simulink subsystem "Doublet"  (R2025a)
settings: Solver=VariableStepAuto  StartTime=0.0  StopTime=10.0  RelTol=1e-3
settings Model: Creator=17036  LastModifiedBy=gurt1

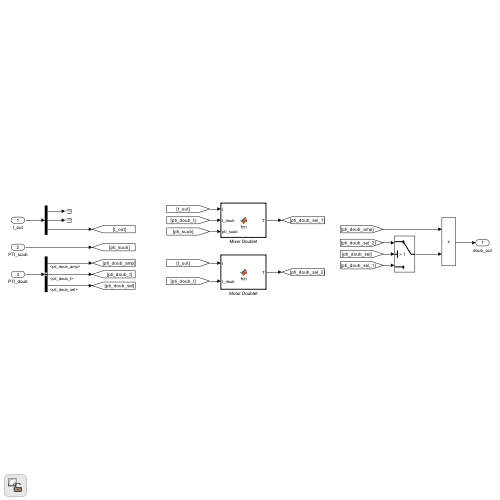
[thumbnail: Simulink's stored preview of the top-level diagram]
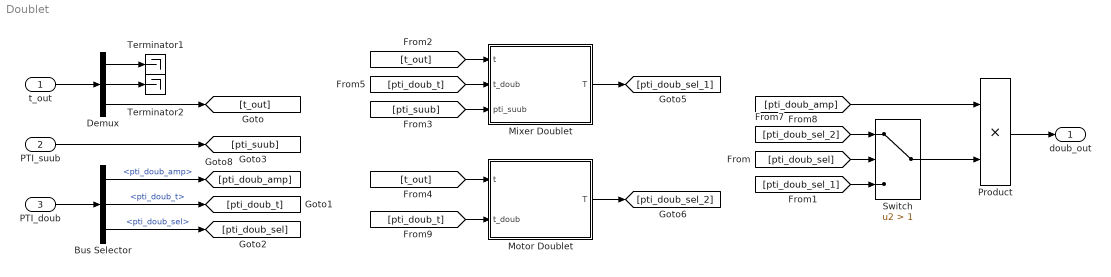
== system Doublet ==
  t_out : Inport
  PTI_suub : Inport  Port=2
  PTI_doub : Inport  Port=3
  Bus Selector : BusSelector  OutputSignals=pti_doub_amp,pti_doub_t,pti_doub_sel
  Demux : Demux  Outputs=3
  Mixer Doublet : MATLAB Function  TreatAsAtomicUnit=on
  Motor Doublet : MATLAB Function  TreatAsAtomicUnit=on
  Product : Product
  Switch : Switch  Criteria=u2 > Threshold  Threshold=1  SaturateOnIntegerOverflow=off  InputSameDT=off
  Terminator1 : Terminator
  Terminator2 : Terminator
  doub_out : Outport
  wires:
  PTI_doub/1 -> Bus Selector/1
  Bus Selector/1 -> [pti_doub_amp]  "<pti_doub_amp>"
  Bus Selector/2 -> [pti_doub_t]  "<pti_doub_t>"
  Bus Selector/3 -> [pti_doub_sel]  "<pti_doub_sel>"
  [pti_doub_sel] -> Switch/2
  Mixer Doublet/1(T) -> [pti_doub_sel_1]
  [t_out] -> Mixer Doublet/1(t)
  Switch/1 -> Product/2
  [pti_doub_amp] -> Product/1
  Product/1 -> doub_out/1
  t_out/1 -> Demux/1
  Motor Doublet/1(T) -> [pti_doub_sel_2]
  PTI_suub/1 -> [pti_suub]
  [pti_doub_t] -> Mixer Doublet/2(t_doub)
  [pti_suub] -> Mixer Doublet/3(pti_suub)
  [pti_doub_t] -> Motor Doublet/2(t_doub)
  [t_out] -> Motor Doublet/1(t)
  Demux/2 -> Terminator2/1
  [pti_doub_sel_2] -> Switch/1
  [pti_doub_sel_1] -> Switch/3
  Demux/3 -> [t_out]
  Demux/1 -> Terminator1/1

== matlab function Doublet/Mixer Doublet ==
  data: t input; T output; t_doub input; pti_suub input
function T = fcn(t, t_doub, pti_suub)

% Roll, Pitch, Yaw, Thrust

% Mixing matrix for quadcopter control (roll, pitch, yaw, throttle)
M = [-1  1 -1 1;
      1 -1 -1 1;
      1  1  1 1;
     -1 -1  1 1];

% Select the column corresponding to the axis mode
axis_mode = M(:,pti_suub+1);

% Calculate the total duration of one full 1-2-1 doublet cycle
cycle_t = 4 * t_doub;

% Find the current time within the current cycle
% current_cycle_t = mod(t, cycle_t);

% Determine the control input based on the time within the cycle
if t>0

if t < t_doub
    % First 1x input
    T = axis_mode;
elseif t < 3 * t_doub
    % 2x input
    T = -1 .* axis_mode;
elseif t < 4 * t_doub
    % Second 1x input
    T = axis_mode;
else
    % Default or zero input
    T = zeros(4, 1);
end

else
    T = zeros(4, 1);
end

== matlab function Doublet/Motor Doublet ==
  data: t input; T output; t_doub input
function T = fcn(t, t_doub)

T = zeros(4,1);
if t > 0
    sequence = [1, -1, 0];
    idx = mod(floor(t/t_doub),12);
    T_idx = floor(idx/3);

    if T_idx<4
        T(T_idx+1) = sequence(mod(idx,3)+1);
    end
end
